simulink model "MPCcreation"  (R2016a)
settings: Solver=ode45  StartTime=0.0  StopTime=3000  RelTol=1e-3
StartFcn:
  | % clear all
  | load('choosed_models');
undefined symbols (not defined in the file or in its folder): model_arx, model_bj, model_oe, model_tf
libraries: slident x6, mpclib x1
settings Model: Creator=johnh  LastModifiedBy=tiago
settings DataIOCC: SaveFormat=StructureWithTime
settings OptimizationCC: BlockReduction=off  DefaultParameterBehavior=Inlined  BufferReuse=off
settings HardwareCC: ProdWordSize=32  ProdHWDeviceType=Specified
settings ConfigComp: CovModelRefEnable=Off

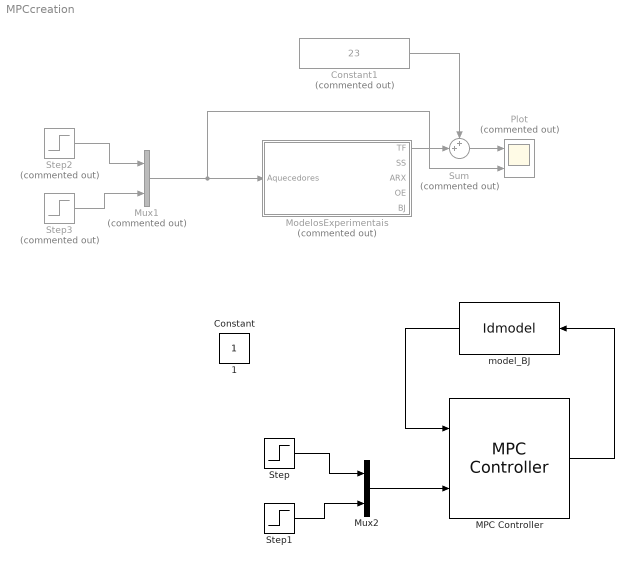
== system MPCcreation ==
  Constant1 : Constant  Commented=on  Value=23
  MPC Controller : mpclib/MPC Controller  SCDEnableBlockLinearizationSpecification=on  is_multiple=0  enable_value=0  return_u0=off  ref_from_ws=off  ref_signal_name=[]  ref_preview=off  md_from_ws=off  md_signal_name=[]  md_preview=off  from_project=off  project_file=MPCtask.mat  md_inport=off  mv_inport=off  cost_outport=off  return_sequence=off  return_qpstatus=off  return_state=off  state_inport=off  lims_inport=off  ywt_inport=off  is_designfromscratch=0  uwt_inport=off  duwt_inport=off  rhoeps_inport=off  uref_inport=off  n_ts=7  n_mv=2  n_md=0  n_ud=0  n_mo=2  n_uo=0  BlockDataType=double  SampleTimeInherited=off  switch_inport=off
  ModelosExperimentais : Subsystem  Commented=on
  Mux1 : Mux  Commented=on  Inputs=2
  Mux2 : Mux  Inputs=2
  Plot : Scope  Commented=on  NumInputPorts=2
  Step : Step  After=50  SampleTime=0
  Step1 : Step  After=40  SampleTime=0
  Step2 : Step  Commented=on  After=50  SampleTime=0
  Step3 : Step  Commented=on  Time=500  After=70  SampleTime=0
  Sum : Sum  Commented=on  Inputs=++|
  model_BJ : slident/Models/Idmodel  sys=model_bj.model{1,1}  IC=0  noi=on  seed=[]
  1 : Constant  IOType=siggen
  Constant : Constant  IOType=siggen
  wires:
  Step/1 -> Mux2/1
  Step1/1 -> Mux2/2
  MPC Controller/1 -> model_BJ/1
  model_BJ/1 -> MPC Controller/1
  Mux2/1 -> MPC Controller/2
  Step2/1 -> Mux1/1
  Step3/1 -> Mux1/2
  Constant1/1 -> Sum/1
  Sum/1 -> Plot/1
  Mux1/1 -> ModelosExperimentais/1(Aquecedores), Plot/2
  ModelosExperimentais/1(TF) -> Sum/2

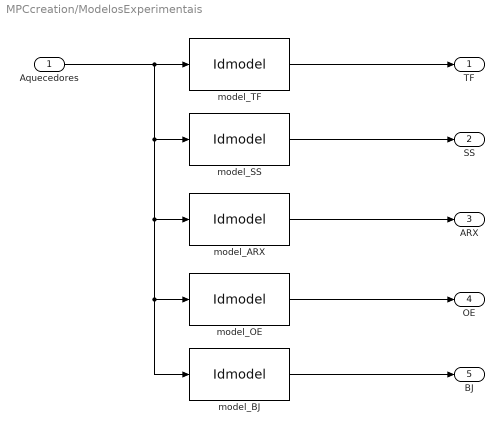
== system MPCcreation/ModelosExperimentais ==
  Aquecedores : Inport
  model_ARX : slident/Models/Idmodel  sys=model_arx.model{1,1}  IC=0  noi=on  seed=[]
  model_BJ : slident/Models/Idmodel  sys=model_bj.model{1,1}  IC=0  noi=on  seed=[]
  model_OE : slident/Models/Idmodel  sys=model_oe.model{1,1}  IC=0  noi=on  seed=[]
  model_SS : slident/Models/Idmodel  sys=model_ss  IC=0  noi=on  seed=[]
  model_TF : slident/Models/Idmodel  sys=model_tf.model{1,1}  IC=0  noi=on  seed=[]
  TF : Outport
  SS : Outport  Port=2
  ARX : Outport  Port=3
  OE : Outport  Port=4
  BJ : Outport  Port=5
  wires:
  Aquecedores/1 -> model_BJ/1, model_OE/1, model_ARX/1, model_SS/1, model_TF/1
  model_TF/1 -> TF/1
  model_SS/1 -> SS/1
  model_ARX/1 -> ARX/1
  model_OE/1 -> OE/1
  model_BJ/1 -> BJ/1
